simulink model "IKS02A1_VL53L8A1_Both"  (R2024b)
settings: Solver=FixedStepDiscrete  StartTime=0.0  StopTime=inf  RelTol=1e-3  EnableMultiTasking=on
PreLoadFcn:
  | addpath(genpath(pwd))
InitFcn:
  | addpath(genpath(pwd));
  | auto_program("IKS02A1_VL53L8A1_Both");
  | STLINK_COMPORT = auto_COMPORT()
  | 
  | dialogPrms = get_param(gcs+"/ISM330DHCX", 'DialogParameters');
  | dialogPrmNames = fieldnames(dialogPrms);
  | odr1 = get_param(gcs+"/ISM330DHCX", dialogPrmNames{2});
  | odr2 = get_param(gcs+"/ISM330DHCX", dialogPrmNames{4});
  | odr1 = eval(odr1);
  | odr2 = eval(odr2);
  | 
  | dialogPrms = get_param(gcs+"/IIS2DLPC", 'DialogParameters');
  | dialogPrmNames = fieldnames(dialogPrms);
  | odr3 = get_param(gcs+"/IIS2DLPC", dialogPrmNames{2});
  | odr3 = eval(odr3);
  | 
  | dialogPrms = get_param(gcs+"/IIS2MDC", 'DialogParameters');
  | dialogPrmNames = fieldnames(dialogPrms);
  | odr4 = get_param(gcs+"/IIS2MDC", dialogPrmNames{1});
  | odr4 = eval(odr4);
  | 
  | dialogPrms = get_param(gcs+"/VL53L8A1", 'DialogParameters');
  | dialogPrmNames = fieldnames(dialogPrms);
  | odr5 = get_param(gcs+"/VL53L8A1", dialogPrmNames{1});
  | odr5 = eval(odr5);
  | 
  | STM32_ODR = max([odr1 odr2 odr3 odr4 odr5])
  | clearvars -except STLINK_COMPORT STLINK_DRIVE STM32_ODR
libraries: etargetslib x14, instrumentseriallib x3
settings Model: SimulationMode=accelerator  PacingRate=0.100000  ExtModeTrigDuration=10  Creator=JesseJabezArendse  LastModifiedBy=JesseJabezArendse
settings OptimizationCC: ReuseModelBlockBuffer=off  PassReuseOutputArgsAs=Individual arguments  ZeroExternalMemoryAtStartup=off  ZeroInternalMemoryAtStartup=off  MaxStackSize=64  OptimizationLevel=level1  OptimizationCustomize=off  EfficientTunableParamExpr=on
settings DebuggingCC: ParameterPrecisionLossMsg=none  ParameterTunabilityLossMsg=error  UnderSpecifiedDimensionMsg=warning
settings HardwareCC: ProdBitPerPointer=32  ProdBitPerSizeT=32  ProdBitPerPtrDiffT=32  ProdLargestAtomicInteger=Long  ProdLargestAtomicFloat=Double  ProdWordSize=32  ProdLongLongMode=on  ProdHWDeviceType=ARM Compatible->ARM Cortex
settings ModelReferenceCC: EnableParallelModelReferenceBuilds=on
settings SFSimCC: SimCustomHeaderCode="#include \"Core\\Inc\\main.h\""  SimParseCustomCode=off  MATLABDynamicMemAlloc=off  SimHardwareAcceleration=native
settings SFSimCC: SimUserSources=|
  | Core\Src\main.c
  | Core\Src\IKS02A1_Simulink.c
settings SFSimCC: SimUserIncludeDirs=|
  | Core\Inc\
  | Core\Src\
settings RTWCC: Description=Embedded Coder  SystemTargetFile=ert.tlc  TemplateMakefile=ert_default_tmf  RTWUseSimCustomCode=on  CustomHeaderCode="#include \"Core\\Inc\\main.h\""  Toolchain=GNU Tools for ARM Embedded Processors  BuildConfiguration=Specify  GPUComputeCapability=3.5
settings RTWCC: CustomInclude=|
  | Core\Inc\
  | Core\Src\
settings RTWCC: CustomSource=|
  | Core\Src\main.c
  | Core\Src\IKS02A1_Simulink.c
settings CodeAppCC: ForceParamTrailComments=on  IgnoreCustomStorageClasses=off  OperatorAnnotations=on  SimulinkDataObjDesc=on  SFDataObjDesc=on  InsertBlockDesc=on
settings ERTTargetCC: CodeReplacementLibrary=ARM Cortex-M  SupportContinuousTime=on  ExtModeTransport=3  ExtModeStaticAlloc=on  ExtModeStaticAllocSize=2000  ExtModeMexFile=ext_xcp  ExtModeIntrfLevel=Level2 - Open  InlinedParameterPlacement=Hierarchical  ERTCustomFileTemplate=example_file_process.tlc  DynamicArrayContainerType=coder::array

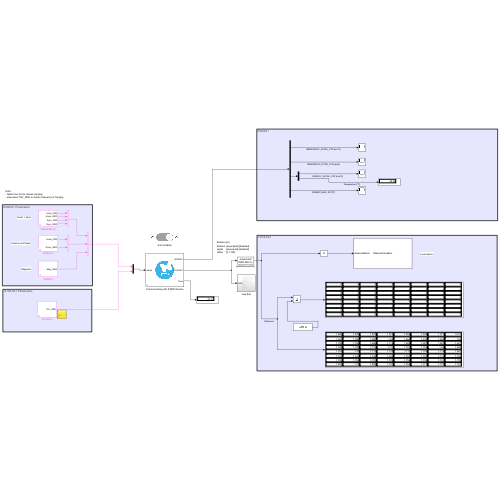
[thumbnail: Simulink's stored preview of the top-level diagram]
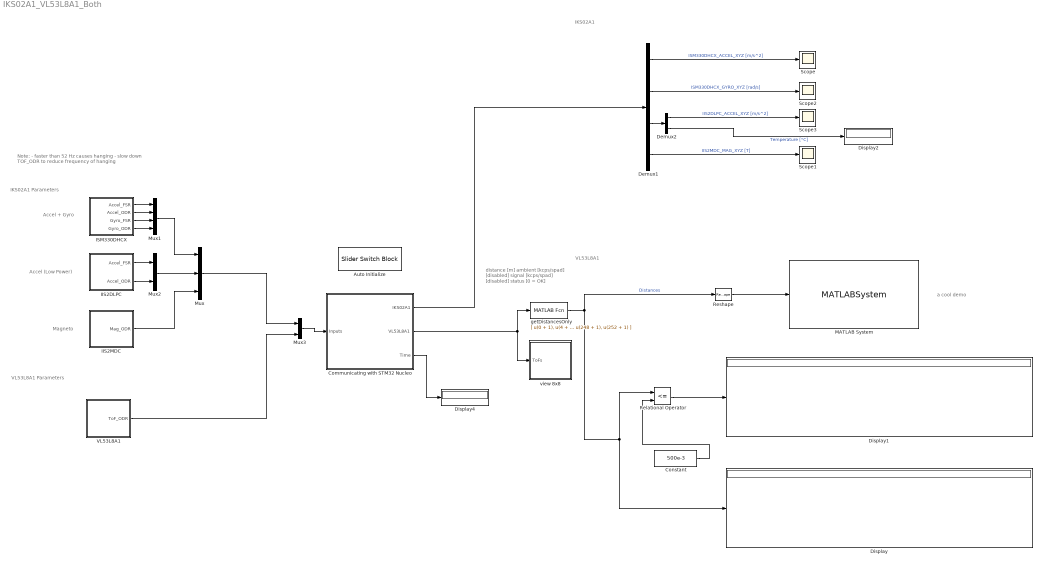
== system IKS02A1_VL53L8A1_Both ==
  note: a cool demo
  note: IKS02A1
  note: VL53L8A1
  note: Note:
      | - faster than 52 Hz causes hanging
      | - slow down TOF_ODR to reduce frequency of hanging
  note: VL53L8A1 Parameters
  note: distance [m]
      | ambient [kcps/spad] [disabled]
      | signal [kcps/spad] [disabled]
      | status [0 = OK]
  note: Accel (Low Power)
  note: Accel + Gyro
  note: Magneto
  note: IKS02A1 Parameters
  Auto Initialize : SliderSwitchBlock  LabelPosition=Hide
      settings: Values={{'Off', 'On'}, [0 1]}
  Communicating with STM32 Nucleo : Subsystem  mask{Auto_Initialize=1}
      mask prompts: Auto_Initialize "Automate Initialization?"
      mask TypeOptions Auto_Initialize: 1 | 0
      mask DialogControl Control1 Prompt: Block for communication between host machine and STM32 Nucleo F411RE
      mask Display: image('stm32_icon.png', [0,0,0,0,80,80]);
  Constant : Constant  Value=500e-3
  Demux1 : Demux  Outputs=[3 3 4 3]
  Demux2 : Demux  Outputs=[3 1]
  Display{,1..2,4} (4 alike) : Display
  IIS2DLPC : Subsystem  mask{FSR_AccelOption=16, ODR_AccelOption=50}
      mask prompts: FSR_AccelOption "Full Scale Range (g)"; ODR_AccelOption "Output Data Rate (Hz)"
      mask init:
      | FSR_AccelVals = [2, 4, 8, 16];
      |     FSR_AccelVal = FSR_AccelVals(FSR_AccelOption);
      |     
      |     ODR_AccelVals = [0 , 1.6 , 12.5 , 25 , 50 , 100 , 200 , 400 , 800 , 1600];
      |     ODR_AccelVal = ODR_AccelVals(ODR_AccelOption);
      mask TypeOptions FSR_AccelOption: 2 | 4 | 8 | 16
      mask TypeOptions ODR_AccelOption: 0 | 1.6 | 12.5 | 25 | 50 | 100 | 200 | 400 | 800 | 1600
      mask DialogControl DescGroupVar Prompt: Accelerometer
  IIS2MDC : Subsystem  mask{ODR_MagOption=50}
      mask prompts: ODR_MagOption "Output Data Rate (Hz)"
      mask init:
      | ODR_MagVals = [10 , 20 , 50 , 100];
      |     ODR_MagVal = ODR_MagVals(ODR_MagOption);
      mask TypeOptions ODR_MagOption: 10 | 20 | 50 | 100
      mask DialogControl DescGroupVar Prompt: Magnetometer
  ISM330DHCX : Subsystem  mask{FSR_AccelOption=16, ODR_AccelOption=52, FSR_GyroOption=4000, ODR_GyroOption=52}
      mask prompts: FSR_AccelOption "Full Scale Range (g)"; ODR_AccelOption "Output Data Rate (Hz)"; FSR_GyroOption "Full Scale Range (dps)"; ODR_GyroOption "Output Data Rate (Hz)"
      mask init:
      | FSR_AccelVals = [2, 4, 8, 16];
      |     FSR_AccelVal = FSR_AccelVals(FSR_AccelOption);
      |     
      |     ODR_AccelVals = [0 , 12.5 , 16 , 52 , 104 , 208 , 416 , 833 , 1666 , 3332 , 6667];
      |     ODR_AccelVal = ODR_AccelVals(ODR_AccelOption);
      | 
      |     FSR_GyroVals = [125, 250, 500, 1000, 2000, 4000];
      |     FSR_GyroVal = FSR_GyroVals(FSR_GyroOption);
      | 
      |     ODR_GyroVals = [0 , 12.5 , 16 , 52 , 104 , 208 , 416 , 833 , 1666 , 3332 , 6667];
      |     ODR_GyroVal = ODR_GyroVals(ODR_GyroOption);
      mask TypeOptions FSR_AccelOption: 2 | 4 | 8 | 16
      mask TypeOptions ODR_AccelOption: 0 | 12.5 | 16 | 52 | 104 | 208 | 416 | 833 | 1666 | 3332 | 6667
      mask TypeOptions FSR_GyroOption: 125 | 250 | 500 | 1000 | 2000 | 4000
      mask TypeOptions ODR_GyroOption: 0 | 12.5 | 16 | 52 | 104 | 208 | 416 | 833 | 1666 | 3332 | 6667
      mask DialogControl DescGroupVar Prompt: Accelerometer
      mask DialogControl DescGroupVar_copy Prompt: Gyroscope
  MATLAB System : MATLABSystem  System=DistanceVisualizer
      mask Type: DistanceVisualizer
      mask Display:
      | disp('DistanceVisualizer');
      | port_label('input',1,'distanceMatrix');
  Mux : Mux  Inputs=3
  Mux1 : Mux
  Mux2 : Mux  Inputs=2
  Mux3 : Mux  Inputs=2
  Relational Operator : RelationalOperator  Operator=<=  OutDataTypeStr=boolean  RndMeth=Simplest  InputSameDT=off
  Reshape : Reshape  OutputDimensionality=Customize  OutputDimensions=[8 , 8]
  Scope{,1..3} (4 alike) : Scope
  VL53L8A1 : Subsystem  mask{ODR_TOF=20.0}
      mask prompts: ODR_TOF "Output Data Rate (Hz)"
      mask DialogControl DescGroupVar Prompt: Time of Flight Sensor 8x8
  getDistancesOnly : MATLABFcn  MATLABFcn=|  OutputDimensions=[64]
      | [ u(0 + 1),
      | u(4 + 1),
      | u(8 + 1),
      | u(12 + 1),
      | u(16 + 1),
      | u(20 + 1),
      | u(24 + 1),
      | u(28 + 1),
      | u(32 + 1),
      | u(36 + 1),
      | u(40 + 1),
      | u(44 + 1),
      | u(48 + 1),
      | u(52 + 1),
      | u(56 + 1),
      | u(60 + 1),
      | u(64 + 1),
      | u(68 + 1),
      | u(72 + 1),
      | u(76 + 1),
      | u(80 + 1),
      | u(84 + 1),
      | u(88 + 1),
      | u(92 + 1),
      | u(96 + 1),
      | u(100 + 1),
      | u(104 + 1),
      | u(108 + 1),
      | u(112 + 1),
      | u(116 + 1),
      | u(120 + 1),
      | u(124 + 1),
      | u(128 + 1),
      | u(132 + 1),
      | u(136 + 1),
      | u(140 + 1),
      | u(144 + 1),
      | u(148 + 1),
      | u(152 + 1),
      | u(156 + 1),
      | u(160 + 1),
      | u(164 + 1),
      | u(168 + 1),
      | u(172 + 1),
      | u(176 + 1),
      | u(180 + 1),
      | u(184 + 1),
      | u(188 + 1),
      | u(192 + 1),
      | u(196 + 1),
      | u(200 + 1),
      | u(204 + 1),
      | u(208 + 1),
      | u(212 + 1),
      | u(216 + 1),
      | u(220 + 1),
      | u(224 + 1),
      | u(228 + 1),
      | u(232 + 1),
      | u(236 + 1),
      | u(240 + 1),
      | u(244 + 1),
      | u(248 + 1),
      | u(252 + 1)
      | 
      | ]
  view 8x8 : Subsystem
  wires:
  getDistancesOnly/1 -> Relational Operator/1, Display/1, Reshape/1  "Distances"
  Constant/1 -> Relational Operator/2
  Relational Operator/1 -> Display1/1
  Communicating with STM32 Nucleo/3(Time) -> Display4/1
  Communicating with STM32 Nucleo/2(VL53L8A1) -> getDistancesOnly/1, view 8x8/1(ToFs)
  VL53L8A1/1(ToF_ODR) -> Mux3/2
  Reshape/1 -> MATLAB System/1
  Mux2/1 -> Mux/2
  ISM330DHCX/3(Gyro_FSR) -> Mux1/3
  Mux1/1 -> Mux/1
  Mux/1 -> Mux3/1
  IIS2MDC/1(Mag_ODR) -> Mux/3
  ISM330DHCX/2(Accel_ODR) -> Mux1/2
  IIS2DLPC/1(Accel_FSR) -> Mux2/1
  IIS2DLPC/2(Accel_ODR) -> Mux2/2
  ISM330DHCX/4(Gyro_ODR) -> Mux1/4
  Mux3/1 -> Communicating with STM32 Nucleo/1(Inputs)
  ISM330DHCX/1(Accel_FSR) -> Mux1/1
  Demux2/1 -> Scope3/1  "IIS2DLPC_ACCEL_XYZ [m/s^2]"
  Demux1/3 -> Demux2/1
  Demux1/4 -> Scope1/1  "IIS2MDC_MAG_XYZ [T]"
  Demux2/2 -> Display2/1  "Temperature [°C]"
  Demux1/2 -> Scope2/1  "ISM330DHCX_GYRO_XYZ [rad/s]"
  Demux1/1 -> Scope/1  "ISM330DHCX_ACCEL_XYZ [m/s^2]"
  Communicating with STM32 Nucleo/1(IKS02A1) -> Demux1/1

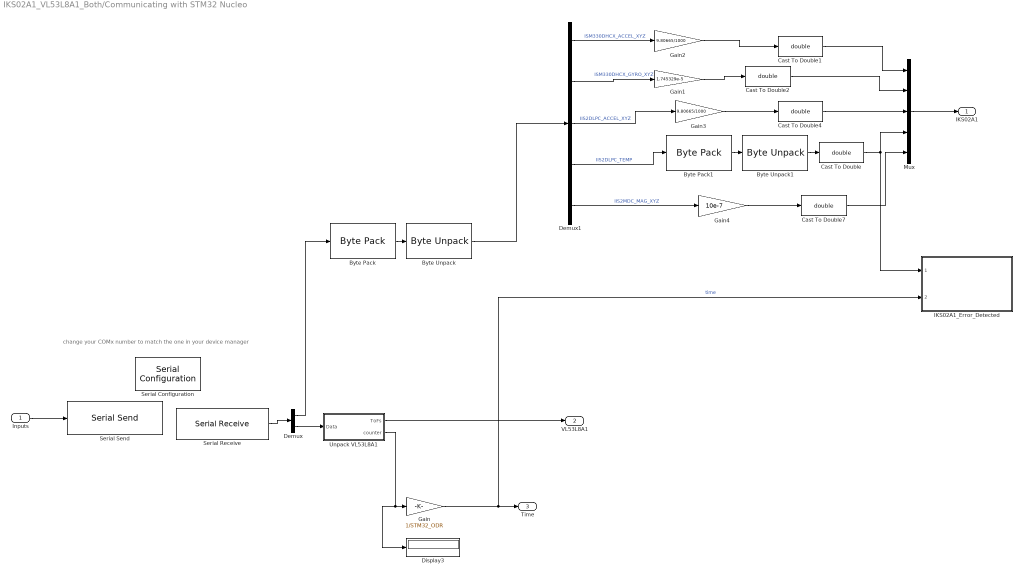
== system IKS02A1_VL53L8A1_Both/Communicating with STM32 Nucleo ==
  note: change your COMx number to match the one in your device manager
  Inputs : Inport
  Byte Pack : etargetslib/Byte Pack  datatypes={'single'}  byteAlign=1
  Byte Pack1 : etargetslib/Byte Pack  datatypes={'int32'}  byteAlign=1
  Byte Unpack : etargetslib/Byte Unpack  dimensions={[13]}  datatypes={'int32'}  byteAlign=1
      settings: LibrarySourceBlock=embeddedtargetslib/Host Communication/Byte Unpack
  Byte Unpack1 : etargetslib/Byte Unpack  dimensions={[1]}  datatypes={'single'}  byteAlign=1
      settings: LibrarySourceBlock=embeddedtargetslib/Host Communication/Byte Unpack
  Cast To Double{,1..2,4,7} (5 alike) : DataTypeConversion  OutDataTypeStr=double  SaturateOnIntegerOverflow=off  RndMeth=Floor
  Demux : Demux  Outputs=[13 257 ]
  Demux1 : Demux  Outputs=[3 3 3 1 3]
  Display3 : Display
  Gain : Gain  Gain=1/STM32_ODR
  Gain1 : Gain  Gain=1.745329e-5
  Gain2 : Gain  Gain=9.80665/1000
  Gain3 : Gain  Gain=9.80665/1000
  Gain4 : Gain  Gain=10e-7
  IKS02A1_Error_Detected : Subsystem  ReferencedSubsystem=IKS02A1_Error_Detected
  Mux : Mux  Inputs=[3 3 3 1 3]
  Serial Configuration : instrumentseriallib/Serial Configuration  Priority=-200000  PortSel=STLINK_COMPORT  Port=STLINK_COMPORT  ComPort=STLINK_COMPORT  BaudRate=1843200  DataBits=8  Parity=even  StopBits=2  ByteOrder=little-endian  FlowControl=none  Timeout=5  SimulateUsing=Interpreted execution  BlockInModel=on  aMode=1
      settings: LibrarySourceBlock=embeddedtargetslib/Host Communication/Serial Configuration
  Serial Receive : instrumentseriallib/Serial Receive  Priority=1  PortSel=STLINK_COMPORT  Port=STLINK_COMPORT  ComPort=STLINK_COMPORT  DataType=single  SaveDataType=uint8  ToggleHeader=on  Header='J_A'  ToggleDataSize=on  DataSize=[1 ((3+3+3+1+3)+ (8*8*4+1))]  ToggleTerminator=on  Terminator=Custom terminator  CustomTerminator='A_J'  InputFormat=Column major  EnableBlockingMode=on  ActionDataUnavailable=Output last received value  ActionWhenDataUnavailable=Output last received value  CustomValue=0  SampleTime=1/STM32_ODR  SimulateUsing=Interpreted execution  BlockInModel=on  aMode=1
      settings: LibrarySourceBlock=embeddedtargetslib/Host Communication/Serial Receive
  Serial Send : instrumentseriallib/Serial Send  Priority=1  PortSel=STLINK_COMPORT  Port=STLINK_COMPORT  ComPort=STLINK_COMPORT  Header='J_A'  Terminator=Custom terminator  CustomTerminator='A_J'  EnableBlockingMode=off  SimulateUsing=Interpreted execution  BlockInModel=on  aMode=1
      settings: LibrarySourceBlock=embeddedtargetslib/Host Communication/Serial Send
  Unpack VL53L8A1 : Subsystem
  IKS02A1 : Outport
  VL53L8A1 : Outport  Port=2
  Time : Outport  Port=3
  wires:
  Demux/2 -> Unpack VL53L8A1/1(Data)
  Gain/1 -> IKS02A1_Error_Detected/2, Time/1  "time"
  Unpack VL53L8A1/1(ToFs) -> VL53L8A1/1
  Unpack VL53L8A1/2(counter) -> Display3/1, Gain/1
  Inputs/1 -> Serial Send/1
  Serial Receive/1 -> Demux/1
  Byte Pack/1 -> Byte Unpack/1
  Demux/1 -> Byte Pack/1
  Demux1/4 -> Byte Pack1/1  "IIS2DLPC_TEMP"
  Demux1/1 -> Gain2/1  "ISM330DHCX_ACCEL_XYZ"
  Cast To Double/1 -> IKS02A1_Error_Detected/1, Mux/4
  Demux1/3 -> Gain3/1  "IIS2DLPC_ACCEL_XYZ"
  Gain1/1 -> Cast To Double2/1
  Gain3/1 -> Cast To Double4/1
  Cast To Double2/1 -> Mux/2
  Byte Unpack/1 -> Demux1/1
  Gain4/1 -> Cast To Double7/1
  Demux1/5 -> Gain4/1  "IIS2MDC_MAG_XYZ"
  Cast To Double1/1 -> Mux/1
  Mux/1 -> IKS02A1/1
  Cast To Double7/1 -> Mux/5
  Demux1/2 -> Gain1/1  "ISM330DHCX_GYRO_XYZ"
  Gain2/1 -> Cast To Double1/1
  Cast To Double4/1 -> Mux/3
  Byte Pack1/1 -> Byte Unpack1/1
  Byte Unpack1/1 -> Cast To Double/1

== system IKS02A1_VL53L8A1_Both/IIS2DLPC ==
  Byte Pack2 : etargetslib/Byte Pack  datatypes={'int32'}  byteAlign=1
  Byte Pack3 : etargetslib/Byte Pack  datatypes={'single'}  byteAlign=1
  Cast4 : DataTypeConversion  OutDataTypeStr=int32  SaturateOnIntegerOverflow=off  RndMeth=Floor
  Cast5 : DataTypeConversion  OutDataTypeStr=single  SaturateOnIntegerOverflow=off  RndMeth=Floor
  Constant : Constant  Value=FSR_AccelVal
  Constant1 : Constant  Value=ODR_AccelVal
  Display : Display
  Display1 : Display
  Accel_FSR : Outport
  Accel_ODR : Outport  Port=2
  wires:
  Constant/1 -> Cast4/1, Display/1
  Constant1/1 -> Cast5/1, Display1/1
  Cast4/1 -> Byte Pack2/1
  Cast5/1 -> Byte Pack3/1
  Byte Pack2/1 -> Accel_FSR/1
  Byte Pack3/1 -> Accel_ODR/1

== system IKS02A1_VL53L8A1_Both/IIS2MDC ==
  Byte Pack3 : etargetslib/Byte Pack  datatypes={'single'}  byteAlign=1
  Cast5 : DataTypeConversion  OutDataTypeStr=single  SaturateOnIntegerOverflow=off  RndMeth=Floor
  Constant1 : Constant  Value=ODR_MagVal
  Display1 : Display
  Mag_ODR : Outport
  wires:
  Constant1/1 -> Cast5/1, Display1/1
  Cast5/1 -> Byte Pack3/1
  Byte Pack3/1 -> Mag_ODR/1

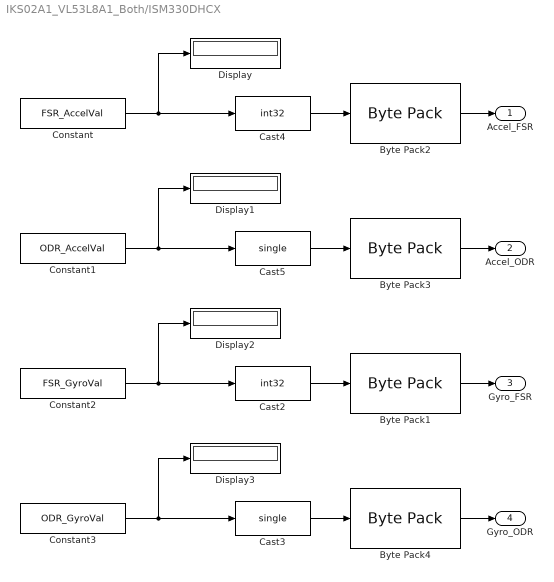
== system IKS02A1_VL53L8A1_Both/ISM330DHCX ==
  Byte Pack1 : etargetslib/Byte Pack  datatypes={'int32'}  byteAlign=1
  Byte Pack2 : etargetslib/Byte Pack  datatypes={'int32'}  byteAlign=1
  Byte Pack3 : etargetslib/Byte Pack  datatypes={'single'}  byteAlign=1
  Byte Pack4 : etargetslib/Byte Pack  datatypes={'single'}  byteAlign=1
  Cast2 : DataTypeConversion  OutDataTypeStr=int32  SaturateOnIntegerOverflow=off  RndMeth=Floor
  Cast3 : DataTypeConversion  OutDataTypeStr=single  SaturateOnIntegerOverflow=off  RndMeth=Floor
  Cast4 : DataTypeConversion  OutDataTypeStr=int32  SaturateOnIntegerOverflow=off  RndMeth=Floor
  Cast5 : DataTypeConversion  OutDataTypeStr=single  SaturateOnIntegerOverflow=off  RndMeth=Floor
  Constant : Constant  Value=FSR_AccelVal
  Constant1 : Constant  Value=ODR_AccelVal
  Constant2 : Constant  Value=FSR_GyroVal
  Constant3 : Constant  Value=ODR_GyroVal
  Display{,1..3} (4 alike) : Display
  Accel_FSR : Outport
  Accel_ODR : Outport  Port=2
  Gyro_FSR : Outport  Port=3
  Gyro_ODR : Outport  Port=4
  wires:
  Constant/1 -> Cast4/1, Display/1
  Constant1/1 -> Cast5/1, Display1/1
  Constant2/1 -> Cast2/1, Display2/1
  Constant3/1 -> Cast3/1, Display3/1
  Cast4/1 -> Byte Pack2/1
  Cast5/1 -> Byte Pack3/1
  Cast2/1 -> Byte Pack1/1
  Cast3/1 -> Byte Pack4/1
  Byte Pack2/1 -> Accel_FSR/1
  Byte Pack3/1 -> Accel_ODR/1
  Byte Pack1/1 -> Gyro_FSR/1
  Byte Pack4/1 -> Gyro_ODR/1

== system IKS02A1_VL53L8A1_Both/VL53L8A1 ==
  Byte Pack3 : etargetslib/Byte Pack  datatypes={'single'}  byteAlign=1
  Cast5 : DataTypeConversion  OutDataTypeStr=single  SaturateOnIntegerOverflow=off  RndMeth=Floor
  Constant1 : Constant  Value=ODR_TOF
  Display1 : Display
  ToF_ODR : Outport
  wires:
  Constant1/1 -> Cast5/1, Display1/1
  Cast5/1 -> Byte Pack3/1
  Byte Pack3/1 -> ToF_ODR/1

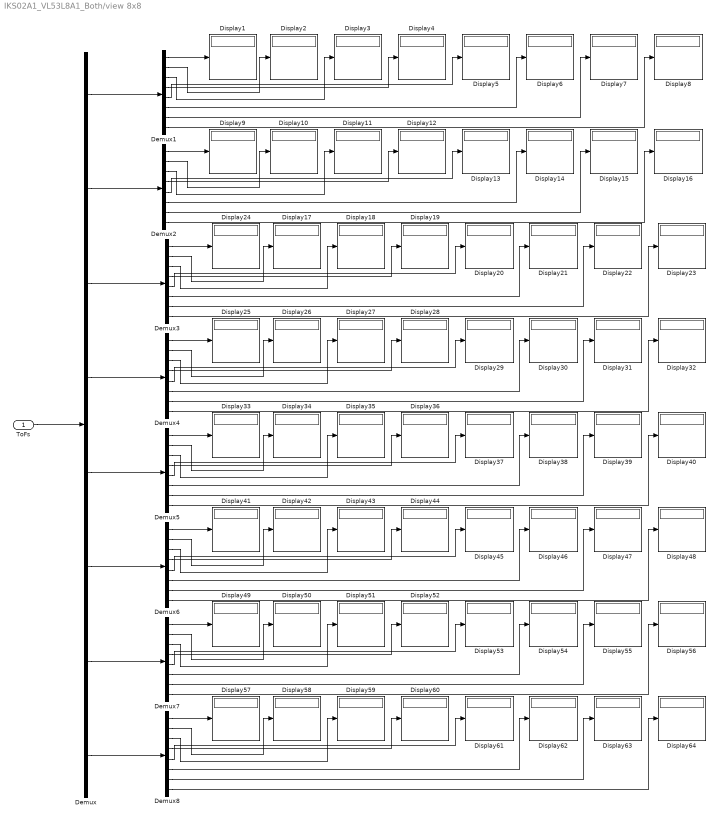
== system IKS02A1_VL53L8A1_Both/view 8x8 ==
  ToFs : Inport
  Demux : Demux  Outputs=[4*8 4*8 4*8 4*8 4*8 4*8 4*8 4*8]
  Demux{1..8} (8 alike) : Demux  Outputs=[4 4 4 4 4 4 4 4]
  Display{1..64} (64 alike) : Display
  wires:
  Demux5/7 -> Display39/1
  Demux4/2 -> Display26/1
  Demux3/3 -> Display18/1
  Demux8/6 -> Display62/1
  Demux3/2 -> Display17/1
  Demux2/2 -> Display10/1
  Demux/5 -> Demux5/1
  Demux1/5 -> Display5/1
  Demux4/4 -> Display28/1
  Demux4/7 -> Display31/1
  Demux4/6 -> Display30/1
  Demux7/7 -> Display55/1
  Demux3/4 -> Display19/1
  Demux/8 -> Demux8/1
  Demux4/8 -> Display32/1
  Demux/4 -> Demux4/1
  Demux8/8 -> Display64/1
  Demux8/3 -> Display59/1
  Demux3/8 -> Display23/1
  Demux4/3 -> Display27/1
  Demux6/4 -> Display44/1
  Demux5/1 -> Display33/1
  Demux1/3 -> Display3/1
  Demux3/7 -> Display22/1
  Demux3/6 -> Display21/1
  Demux1/2 -> Display2/1
  Demux3/5 -> Display20/1
  Demux8/2 -> Display58/1
  Demux/1 -> Demux1/1
  Demux3/1 -> Display24/1
  Demux/2 -> Demux2/1
  Demux7/3 -> Display51/1
  Demux2/5 -> Display13/1
  Demux4/1 -> Display25/1
  Demux1/6 -> Display6/1
  Demux1/8 -> Display8/1
  Demux2/3 -> Display11/1
  Demux5/4 -> Display36/1
  Demux7/6 -> Display54/1
  Demux4/5 -> Display29/1
  Demux/6 -> Demux6/1
  Demux/3 -> Demux3/1
  Demux7/5 -> Display53/1
  Demux5/8 -> Display40/1
  Demux8/7 -> Display63/1
  Demux6/7 -> Display47/1
  Demux5/2 -> Display34/1
  Demux1/7 -> Display7/1
  Demux8/4 -> Display60/1
  Demux6/1 -> Display41/1
  Demux5/5 -> Display37/1
  Demux6/3 -> Display43/1
  Demux6/6 -> Display46/1
  Demux6/2 -> Display42/1
  Demux6/5 -> Display45/1
  Demux1/1 -> Display1/1
  Demux6/8 -> Display48/1
  Demux1/4 -> Display4/1
  Demux8/1 -> Display57/1
  Demux5/6 -> Display38/1
  Demux8/5 -> Display61/1
  Demux5/3 -> Display35/1
  Demux2/8 -> Display16/1
  Demux7/4 -> Display52/1
  Demux7/8 -> Display56/1
  Demux7/1 -> Display49/1
  Demux7/2 -> Display50/1
  Demux2/7 -> Display15/1
  Demux2/6 -> Display14/1
  Demux2/1 -> Display9/1
  Demux2/4 -> Display12/1
  Demux/7 -> Demux7/1
  ToFs/1 -> Demux/1

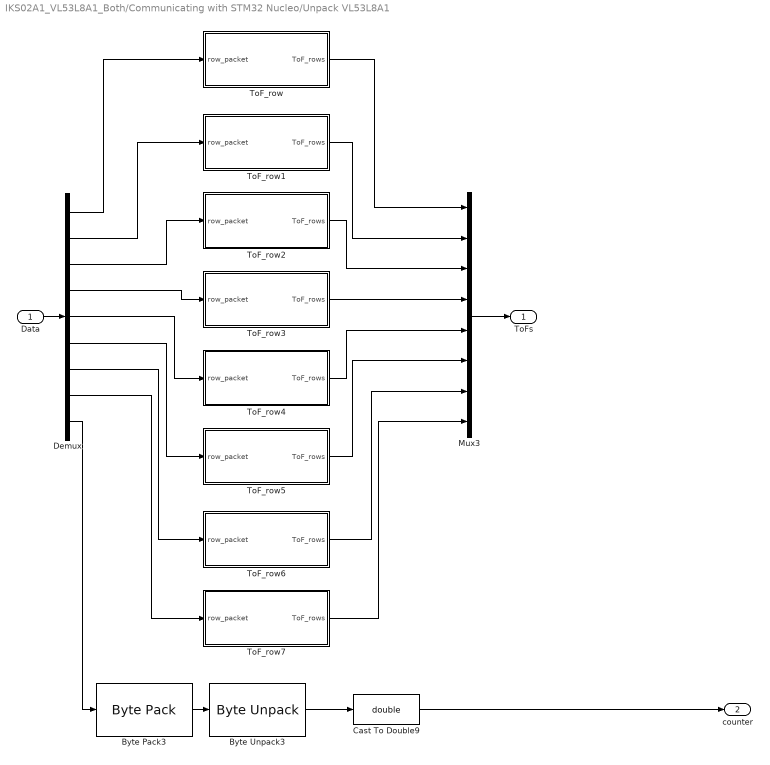
== system IKS02A1_VL53L8A1_Both/Communicating with STM32 Nucleo/Unpack VL53L8A1 ==
  Data : Inport
  Byte Pack3 : etargetslib/Byte Pack  datatypes={'single'}  byteAlign=1
  Byte Unpack3 : etargetslib/Byte Unpack  dimensions={[1]}  datatypes={'uint32'}  byteAlign=1
      settings: LibrarySourceBlock=embeddedtargetslib/Host Communication/Byte Unpack
  Cast To Double9 : DataTypeConversion  OutDataTypeStr=double  SaturateOnIntegerOverflow=off  RndMeth=Floor
  Demux : Demux  Outputs=[4*8 4*8 4*8 4*8 4*8 4*8 4*8 4*8 1]
  Mux3 : Mux  Inputs=[4*8 4*8 4*8 4*8 4*8 4*8 4*8 4*8]
  ToF_row : Subsystem
  ToF_row1 : Subsystem
  ToF_row2 : Subsystem
  ToF_row3 : Subsystem
  ToF_row4 : Subsystem
  ToF_row5 : Subsystem
  ToF_row6 : Subsystem
  ToF_row7 : Subsystem
  ToFs : Outport
  counter : Outport  Port=2
  wires:
  Data/1 -> Demux/1
  Demux/7 -> ToF_row6/1(row_packet)
  Demux/6 -> ToF_row5/1(row_packet)
  Demux/5 -> ToF_row4/1(row_packet)
  Mux3/1 -> ToFs/1
  Demux/4 -> ToF_row3/1(row_packet)
  Demux/3 -> ToF_row2/1(row_packet)
  Demux/2 -> ToF_row1/1(row_packet)
  Demux/1 -> ToF_row/1(row_packet)
  Demux/8 -> ToF_row7/1(row_packet)
  ToF_row/1(ToF_rows) -> Mux3/1
  ToF_row1/1(ToF_rows) -> Mux3/2
  ToF_row2/1(ToF_rows) -> Mux3/3
  ToF_row3/1(ToF_rows) -> Mux3/4
  ToF_row4/1(ToF_rows) -> Mux3/5
  ToF_row5/1(ToF_rows) -> Mux3/6
  ToF_row6/1(ToF_rows) -> Mux3/7
  ToF_row7/1(ToF_rows) -> Mux3/8
  Demux/9 -> Byte Pack3/1
  Byte Unpack3/1 -> Cast To Double9/1
  Cast To Double9/1 -> counter/1
  Byte Pack3/1 -> Byte Unpack3/1

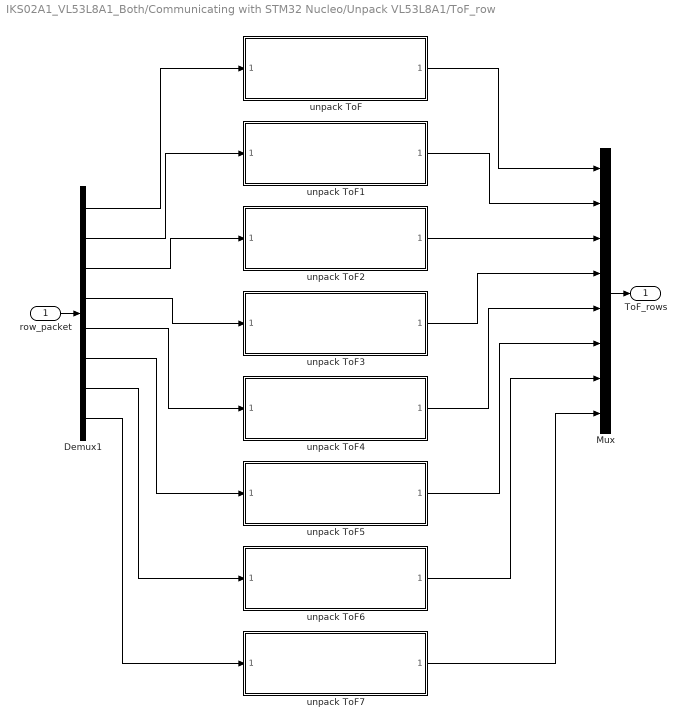
== system IKS02A1_VL53L8A1_Both/Communicating with STM32 Nucleo/Unpack VL53L8A1/ToF_row ==
  row_packet : Inport
  Demux1 : Demux  Outputs=[4 4 4 4 4 4 4 4]
  Mux : Mux  Inputs=[4 4 4 4 4 4 4 4]
  unpack ToF{,1..7} (8 alike) : Subsystem  ReferencedSubsystem=unpack_ToF
  ToF_rows : Outport
  wires:
  Demux1/7 -> unpack ToF6/1
  unpack ToF5/1 -> Mux/6
  unpack ToF3/1 -> Mux/4
  Demux1/1 -> unpack ToF/1
  Demux1/8 -> unpack ToF7/1
  Demux1/3 -> unpack ToF2/1
  Demux1/5 -> unpack ToF4/1
  Demux1/2 -> unpack ToF1/1
  unpack ToF1/1 -> Mux/2
  Demux1/4 -> unpack ToF3/1
  unpack ToF4/1 -> Mux/5
  unpack ToF7/1 -> Mux/8
  Mux/1 -> ToF_rows/1
  Demux1/6 -> unpack ToF5/1
  unpack ToF6/1 -> Mux/7
  unpack ToF/1 -> Mux/1
  unpack ToF2/1 -> Mux/3
  row_packet/1 -> Demux1/1

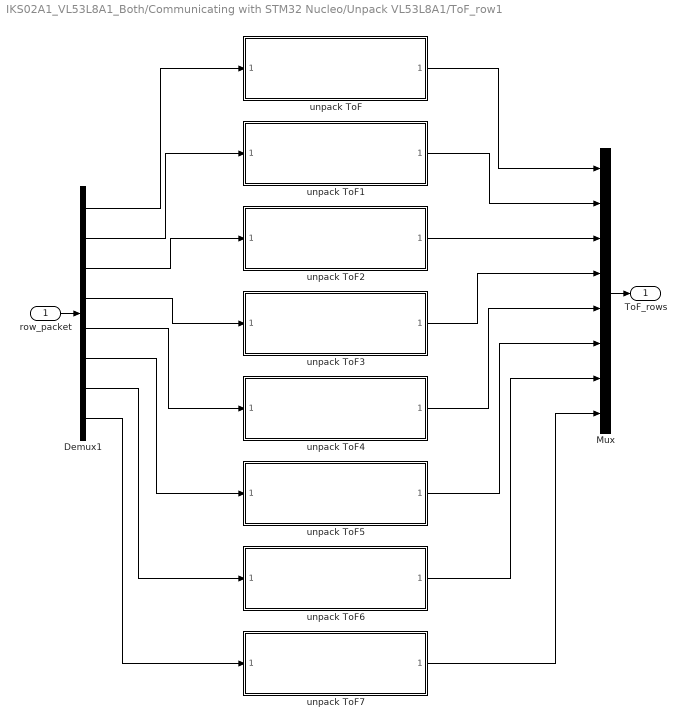
== system IKS02A1_VL53L8A1_Both/Communicating with STM32 Nucleo/Unpack VL53L8A1/ToF_row1 ==
  row_packet : Inport
  Demux1 : Demux  Outputs=[4 4 4 4 4 4 4 4]
  Mux : Mux  Inputs=[4 4 4 4 4 4 4 4]
  unpack ToF{,1..7} (8 alike) : Subsystem  ReferencedSubsystem=unpack_ToF
  ToF_rows : Outport
  wires:
  row_packet/1 -> Demux1/1
  unpack ToF2/1 -> Mux/3
  unpack ToF/1 -> Mux/1
  unpack ToF6/1 -> Mux/7
  Demux1/6 -> unpack ToF5/1
  Mux/1 -> ToF_rows/1
  unpack ToF7/1 -> Mux/8
  unpack ToF4/1 -> Mux/5
  Demux1/4 -> unpack ToF3/1
  unpack ToF1/1 -> Mux/2
  Demux1/2 -> unpack ToF1/1
  Demux1/5 -> unpack ToF4/1
  Demux1/3 -> unpack ToF2/1
  Demux1/8 -> unpack ToF7/1
  Demux1/1 -> unpack ToF/1
  unpack ToF3/1 -> Mux/4
  unpack ToF5/1 -> Mux/6
  Demux1/7 -> unpack ToF6/1

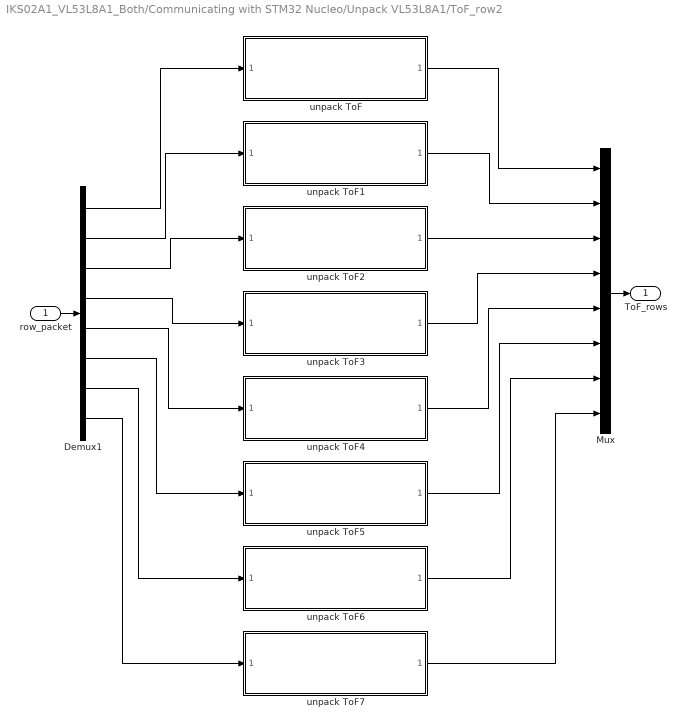
== system IKS02A1_VL53L8A1_Both/Communicating with STM32 Nucleo/Unpack VL53L8A1/ToF_row2 ==
  row_packet : Inport
  Demux1 : Demux  Outputs=[4 4 4 4 4 4 4 4]
  Mux : Mux  Inputs=[4 4 4 4 4 4 4 4]
  unpack ToF{,1..7} (8 alike) : Subsystem  ReferencedSubsystem=unpack_ToF
  ToF_rows : Outport
  wires:
  Demux1/7 -> unpack ToF6/1
  unpack ToF5/1 -> Mux/6
  unpack ToF3/1 -> Mux/4
  Demux1/1 -> unpack ToF/1
  Demux1/8 -> unpack ToF7/1
  Demux1/3 -> unpack ToF2/1
  Demux1/5 -> unpack ToF4/1
  Demux1/2 -> unpack ToF1/1
  unpack ToF1/1 -> Mux/2
  Demux1/4 -> unpack ToF3/1
  unpack ToF4/1 -> Mux/5
  unpack ToF7/1 -> Mux/8
  Mux/1 -> ToF_rows/1
  Demux1/6 -> unpack ToF5/1
  unpack ToF6/1 -> Mux/7
  unpack ToF/1 -> Mux/1
  unpack ToF2/1 -> Mux/3
  row_packet/1 -> Demux1/1

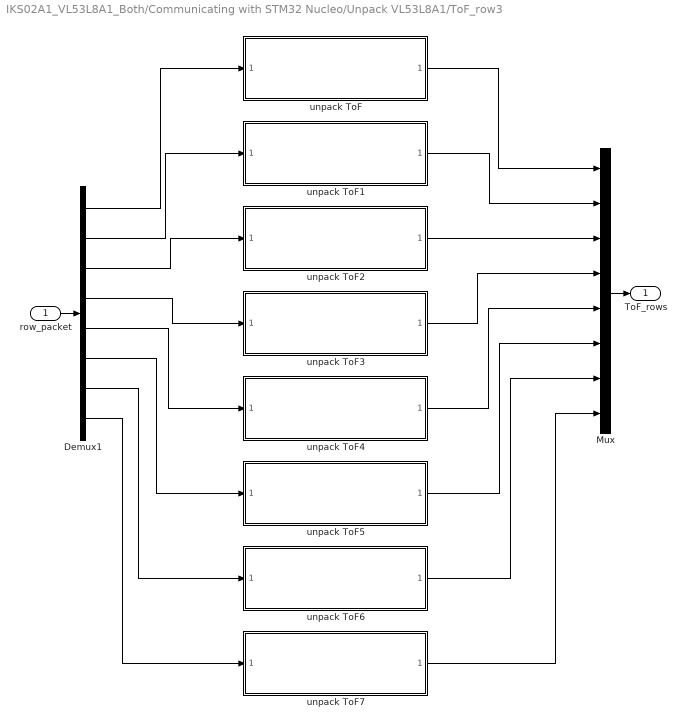
== system IKS02A1_VL53L8A1_Both/Communicating with STM32 Nucleo/Unpack VL53L8A1/ToF_row3 ==
  row_packet : Inport
  Demux1 : Demux  Outputs=[4 4 4 4 4 4 4 4]
  Mux : Mux  Inputs=[4 4 4 4 4 4 4 4]
  unpack ToF{,1..7} (8 alike) : Subsystem  ReferencedSubsystem=unpack_ToF
  ToF_rows : Outport
  wires:
  row_packet/1 -> Demux1/1
  unpack ToF2/1 -> Mux/3
  unpack ToF/1 -> Mux/1
  unpack ToF6/1 -> Mux/7
  Demux1/6 -> unpack ToF5/1
  Mux/1 -> ToF_rows/1
  unpack ToF7/1 -> Mux/8
  unpack ToF4/1 -> Mux/5
  Demux1/4 -> unpack ToF3/1
  unpack ToF1/1 -> Mux/2
  Demux1/2 -> unpack ToF1/1
  Demux1/5 -> unpack ToF4/1
  Demux1/3 -> unpack ToF2/1
  Demux1/8 -> unpack ToF7/1
  Demux1/1 -> unpack ToF/1
  unpack ToF3/1 -> Mux/4
  unpack ToF5/1 -> Mux/6
  Demux1/7 -> unpack ToF6/1

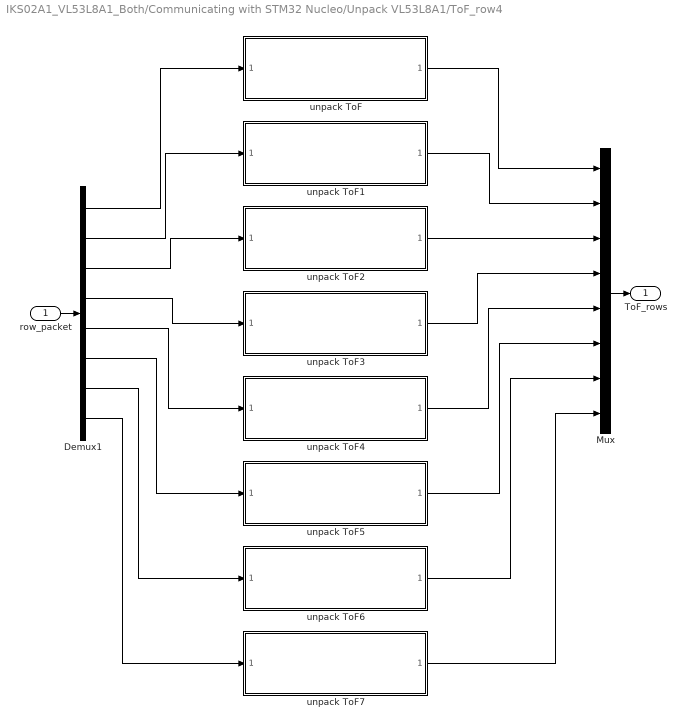
== system IKS02A1_VL53L8A1_Both/Communicating with STM32 Nucleo/Unpack VL53L8A1/ToF_row4 ==
  row_packet : Inport
  Demux1 : Demux  Outputs=[4 4 4 4 4 4 4 4]
  Mux : Mux  Inputs=[4 4 4 4 4 4 4 4]
  unpack ToF{,1..7} (8 alike) : Subsystem  ReferencedSubsystem=unpack_ToF
  ToF_rows : Outport
  wires:
  Demux1/7 -> unpack ToF6/1
  unpack ToF5/1 -> Mux/6
  unpack ToF3/1 -> Mux/4
  Demux1/1 -> unpack ToF/1
  Demux1/8 -> unpack ToF7/1
  Demux1/3 -> unpack ToF2/1
  Demux1/5 -> unpack ToF4/1
  Demux1/2 -> unpack ToF1/1
  unpack ToF1/1 -> Mux/2
  Demux1/4 -> unpack ToF3/1
  unpack ToF4/1 -> Mux/5
  unpack ToF7/1 -> Mux/8
  Mux/1 -> ToF_rows/1
  Demux1/6 -> unpack ToF5/1
  unpack ToF6/1 -> Mux/7
  unpack ToF/1 -> Mux/1
  unpack ToF2/1 -> Mux/3
  row_packet/1 -> Demux1/1

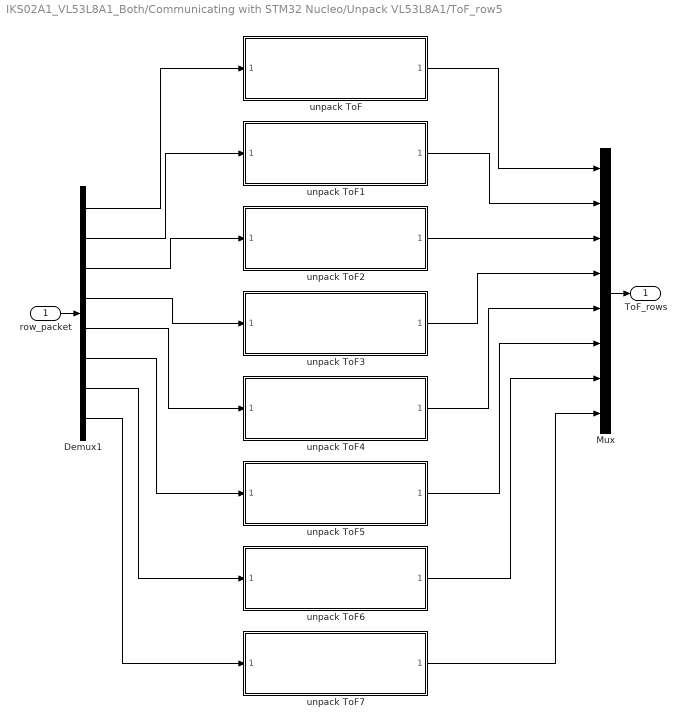
== system IKS02A1_VL53L8A1_Both/Communicating with STM32 Nucleo/Unpack VL53L8A1/ToF_row5 ==
  row_packet : Inport
  Demux1 : Demux  Outputs=[4 4 4 4 4 4 4 4]
  Mux : Mux  Inputs=[4 4 4 4 4 4 4 4]
  unpack ToF{,1..7} (8 alike) : Subsystem  ReferencedSubsystem=unpack_ToF
  ToF_rows : Outport
  wires:
  row_packet/1 -> Demux1/1
  unpack ToF2/1 -> Mux/3
  unpack ToF/1 -> Mux/1
  unpack ToF6/1 -> Mux/7
  Demux1/6 -> unpack ToF5/1
  Mux/1 -> ToF_rows/1
  unpack ToF7/1 -> Mux/8
  unpack ToF4/1 -> Mux/5
  Demux1/4 -> unpack ToF3/1
  unpack ToF1/1 -> Mux/2
  Demux1/2 -> unpack ToF1/1
  Demux1/5 -> unpack ToF4/1
  Demux1/3 -> unpack ToF2/1
  Demux1/8 -> unpack ToF7/1
  Demux1/1 -> unpack ToF/1
  unpack ToF3/1 -> Mux/4
  unpack ToF5/1 -> Mux/6
  Demux1/7 -> unpack ToF6/1

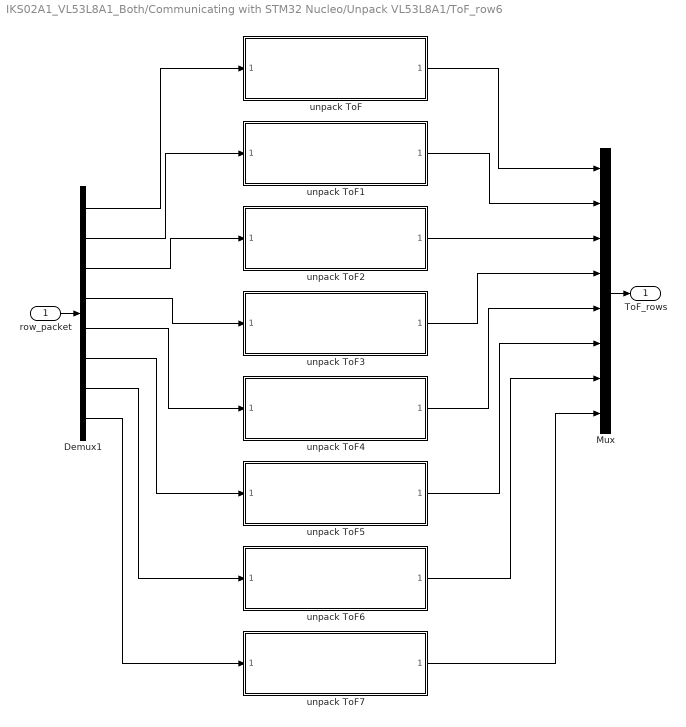
== system IKS02A1_VL53L8A1_Both/Communicating with STM32 Nucleo/Unpack VL53L8A1/ToF_row6 ==
  row_packet : Inport
  Demux1 : Demux  Outputs=[4 4 4 4 4 4 4 4]
  Mux : Mux  Inputs=[4 4 4 4 4 4 4 4]
  unpack ToF{,1..7} (8 alike) : Subsystem  ReferencedSubsystem=unpack_ToF
  ToF_rows : Outport
  wires:
  Demux1/7 -> unpack ToF6/1
  unpack ToF5/1 -> Mux/6
  unpack ToF3/1 -> Mux/4
  Demux1/1 -> unpack ToF/1
  Demux1/8 -> unpack ToF7/1
  Demux1/3 -> unpack ToF2/1
  Demux1/5 -> unpack ToF4/1
  Demux1/2 -> unpack ToF1/1
  unpack ToF1/1 -> Mux/2
  Demux1/4 -> unpack ToF3/1
  unpack ToF4/1 -> Mux/5
  unpack ToF7/1 -> Mux/8
  Mux/1 -> ToF_rows/1
  Demux1/6 -> unpack ToF5/1
  unpack ToF6/1 -> Mux/7
  unpack ToF/1 -> Mux/1
  unpack ToF2/1 -> Mux/3
  row_packet/1 -> Demux1/1

== system IKS02A1_VL53L8A1_Both/Communicating with STM32 Nucleo/Unpack VL53L8A1/ToF_row7 ==
  row_packet : Inport
  Demux1 : Demux  Outputs=[4 4 4 4 4 4 4 4]
  Mux : Mux  Inputs=[4 4 4 4 4 4 4 4]
  unpack ToF{,1..7} (8 alike) : Subsystem  ReferencedSubsystem=unpack_ToF
  ToF_rows : Outport
  wires:
  row_packet/1 -> Demux1/1
  unpack ToF2/1 -> Mux/3
  unpack ToF/1 -> Mux/1
  unpack ToF6/1 -> Mux/7
  Demux1/6 -> unpack ToF5/1
  Mux/1 -> ToF_rows/1
  unpack ToF7/1 -> Mux/8
  unpack ToF4/1 -> Mux/5
  Demux1/4 -> unpack ToF3/1
  unpack ToF1/1 -> Mux/2
  Demux1/2 -> unpack ToF1/1
  Demux1/5 -> unpack ToF4/1
  Demux1/3 -> unpack ToF2/1
  Demux1/8 -> unpack ToF7/1
  Demux1/1 -> unpack ToF/1
  unpack ToF3/1 -> Mux/4
  unpack ToF5/1 -> Mux/6
  Demux1/7 -> unpack ToF6/1
